simulink model "SensorFusion"  (R2024b)
settings: Solver=VariableStepAuto  StartTime=0.0  StopTime=10.0  RelTol=1e-3
libraries: aerolibnav x3, sharedTrackingLibrary x1
settings Model: Creator=rishi  LastModifiedBy=rishi

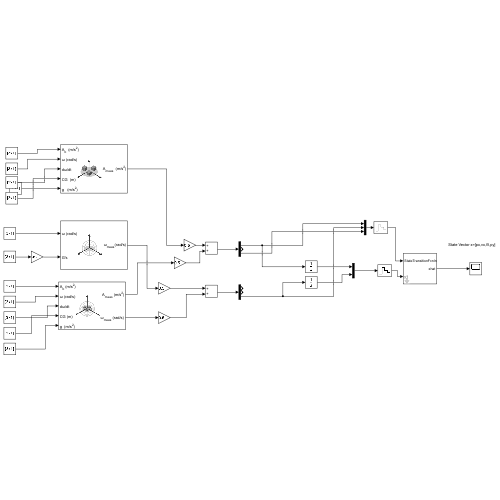
[thumbnail: Simulink's stored preview of the top-level diagram]
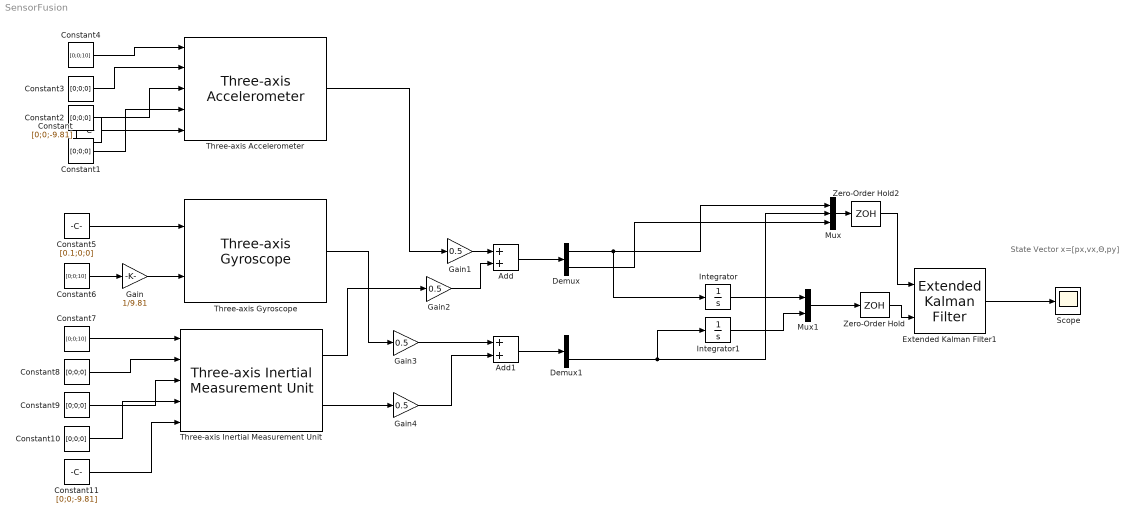
== system SensorFusion ==
  note: State Vector x=[px,vx,Θ,py]
  Add : Sum
  Add1 : Sum
  Constant : Constant  Value=[0;0;-9.81]
  Constant{1..3,8..10} (6 alike) : Constant  Value=[0;0;0]
  Constant11 : Constant  Value=[0;0;-9.81]
  Constant4 : Constant  Value=[0;0;10]
  Constant5 : Constant  Value=[0.1;0;0]
  Constant6 : Constant  Value=[0;0;10]
  Constant7 : Constant  Value=[0;0;10]
  Demux : Demux  Outputs=3
  Demux1 : Demux  Outputs=3
  Extended Kalman Filter1 : sharedTrackingLibrary/Extended Kalman Filter  StateTransitionFcn=stateFcn  HasStateTransitionJacobianFcn=off  HasAdditiveProcessNoise=Additive  ProcessNoise=diag([0.5, 0.5, 0.01, 0.5])  HasTimeVaryingProcessNoise=off  HasStateTransitionFcnExtraArgument=1  InitialState=[0; 0; 0; 0]  InitialStateCovariance=diag([10, 10, 0.1, 10])  MeasurementFcn1=measFcn  HasMeasurementJacobianFcn1=off  HasMeasurementEnablePort1=off  HasAdditiveMeasurementNoise1=Additive  MeasurementNoise1=diag([0.2, 0.01])  HasTimeVaryingMeasurementNoise1=off  HasMeasurementFcnExtraArgument1=0  HasMeasurementWrapping1=off  MeasurementFcn2=measFcn  HasMeasurementJacobianFcn2=off  HasMeasurementEnablePort2=off  HasAdditiveMeasurementNoise2=Additive  MeasurementNoise2=1  HasTimeVaryingMeasurementNoise2=off  HasMeasurementFcnExtraArgument2=0  HasMeasurementWrapping2=off  MeasurementFcn3=myMeasurementFcn  HasMeasurementJacobianFcn3=off  HasMeasurementEnablePort3=off  HasAdditiveMeasurementNoise3=Additive  MeasurementNoise3=1  HasTimeVaryingMeasurementNoise3=off  HasMeasurementFcnExtraArgument3=0  HasMeasurementWrapping3=off  MeasurementFcn4=myMeasurementFcn  HasMeasurementJacobianFcn4=off  HasMeasurementEnablePort4=off  HasAdditiveMeasurementNoise4=Additive  MeasurementNoise4=1  HasTimeVaryingMeasurementNoise4=off  HasMeasurementFcnExtraArgument4=0  HasMeasurementWrapping4=off  MeasurementFcn5=myMeasurementFcn  HasMeasurementJacobianFcn5=off  HasMeasurementEnablePort5=off  HasAdditiveMeasurementNoise5=Additive  MeasurementNoise5=1  HasTimeVaryingMeasurementNoise5=off  HasMeasurementFcnExtraArgument5=0  HasMeasurementWrapping5=off  EnableMultirate=off  StateTransitionFcnSampleTime=1  MeasurementFcn1SampleTime=1  MeasurementFcn2SampleTime=1  MeasurementFcn3SampleTime=1  MeasurementFcn4SampleTime=1  MeasurementFcn5SampleTime=1  UseCurrentEstimator=on  OutputStateCovariance=off  DataType=double  SampleTime=0.01  NumberOfMeasurements=1
  Gain : Gain  Gain=1/9.81
  Gain{1..4} (4 alike) : Gain  Gain=0.5
  Integrator : Integrator
  Integrator1 : Integrator
  Mux : Mux  Inputs=3
  Mux1 : Mux  Inputs=2
  Scope : Scope
  Three-axis Accelerometer : aerolibnav/Three-axis Accelerometer  units=Metric (MKS)  acc=[0 0 0]  gtype=on  dtype_a=on  w_a=190  z_a=0.707  a_sf_cc=[1 0 0; 0 1 0; 0 0 1]  a_bias=[0 0 0]  a_Ts=0  a_rand=on  a_seeds=[23093 23094 23095]  a_pow=[0.001 0.001 0.001]  a_sat="[-inf  -inf  -inf  inf inf inf]"
  Three-axis Gyroscope : aerolibnav/Three-axis Gyroscope  dtype_g=on  w_g=190  z_g=0.707  g_sf_cc=[1 0 0; 0 1 0; 0 0 1]  g_bias=[0 0 0]  g_sen=[0 0 0]  g_Ts=0  g_rand=on  g_seeds=[23093 23094 23095]  g_pow=[0.0001 0.0001 0.0001]  g_sat="[-inf  -inf  -inf  inf inf inf]"
  Three-axis Inertial Measurement Unit : aerolibnav/Three-axis Inertial Measurement Unit  units=Metric (MKS)  imu=[0 0 0]  i_Ts=0  dtype_a=on  w_a=190  z_a=0.707  a_sf_cc=[1 0 0; 0 1 0; 0 0 1]  a_bias=[0 0 0]  a_sat="[-inf  -inf  -inf  inf inf inf]"  dtype_g=on  w_g=190  z_g=0.707  g_sf_cc=[1 0 0; 0 1 0; 0 0 1]  g_bias=[0 0 0]  g_sens=[0 0 0]  g_sat="[-inf  -inf  -inf  inf inf inf]"  i_rand=on  i_seeds=[23093 23094 23095 23096 23097 23098]  i_pow=[0.001 0.001 0.001 0.0001 0.0001 0.0001]
  Zero-Order Hold : ZeroOrderHold  SampleTime=0.01
  Zero-Order Hold2 : ZeroOrderHold  SampleTime=0.01
  wires:
  Constant/1 -> Three-axis Accelerometer/5
  Constant1/1 -> Three-axis Accelerometer/4
  Constant2/1 -> Three-axis Accelerometer/3
  Constant3/1 -> Three-axis Accelerometer/2
  Constant4/1 -> Three-axis Accelerometer/1
  Constant5/1 -> Three-axis Gyroscope/1
  Constant6/1 -> Gain/1
  Gain/1 -> Three-axis Gyroscope/2
  Constant7/1 -> Three-axis Inertial Measurement Unit/1
  Constant8/1 -> Three-axis Inertial Measurement Unit/2
  Constant9/1 -> Three-axis Inertial Measurement Unit/3
  Constant10/1 -> Three-axis Inertial Measurement Unit/4
  Constant11/1 -> Three-axis Inertial Measurement Unit/5
  Three-axis Accelerometer/1 -> Gain1/1
  Three-axis Inertial Measurement Unit/1 -> Gain2/1
  Three-axis Gyroscope/1 -> Gain3/1
  Three-axis Inertial Measurement Unit/2 -> Gain4/1
  Gain1/1 -> Add/1
  Gain2/1 -> Add/2
  Gain3/1 -> Add1/1
  Gain4/1 -> Add1/2
  Add/1 -> Demux/1
  Add1/1 -> Demux1/1
  Demux/1 -> Integrator/1, Mux/1
  Demux1/3 -> Integrator1/1, Mux/2
  Demux/3 -> Mux/3
  Extended Kalman Filter1/1 -> Scope/1
  Mux/1 -> Zero-Order Hold2/1
  Zero-Order Hold/1 -> Extended Kalman Filter1/2
  Zero-Order Hold2/1 -> Extended Kalman Filter1/1
  Integrator/1 -> Mux1/1
  Integrator1/1 -> Mux1/2
  Mux1/1 -> Zero-Order Hold/1
